simulink model "station"  (R2022a)
settings: Solver=VariableStepAuto  StartTime=0.0  StopTime=10.0  RelTol=1e-3
settings Model: Creator=kasturkoul  LastModifiedBy=kasturkoul

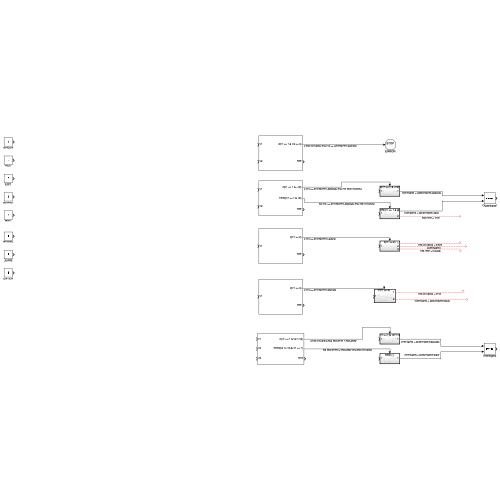
[thumbnail: Simulink's stored preview of the top-level diagram]
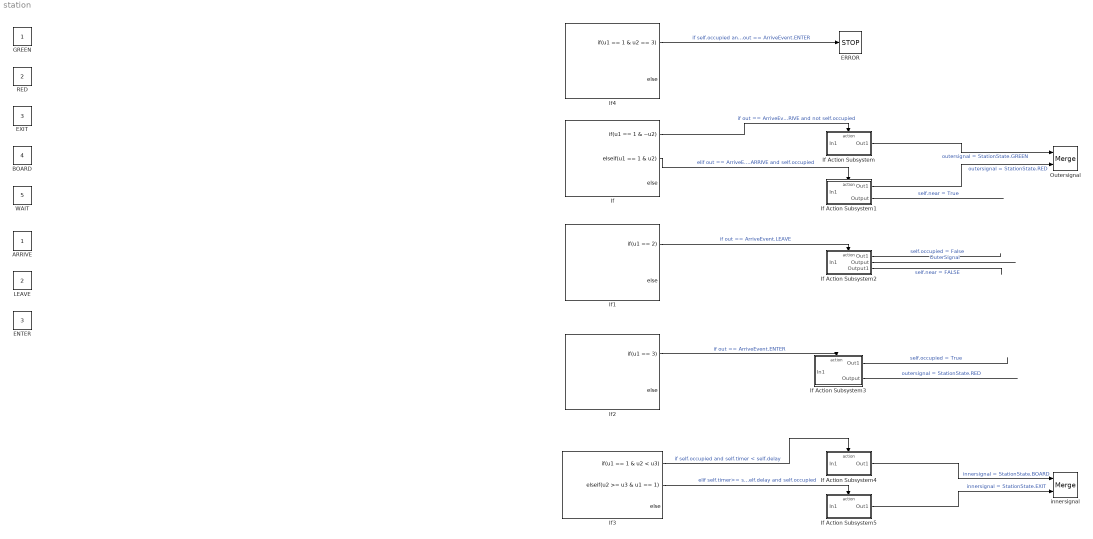
== system station ==
  ARRIVE : Constant
  BOARD : Constant  Value=4
  ENTER : Constant  Value=3
  ERROR : Stop
  EXIT : Constant  Value=3
  GREEN : Constant
  If : If  NumInputs=2  IfExpression=u1 == 1 & ~u2  ElseIfExpressions=u1 == 1 & u2
  If Action Subsystem : Subsystem  TreatAsAtomicUnit=on
  If Action Subsystem1 : Subsystem  TreatAsAtomicUnit=on
  If Action Subsystem2 : Subsystem  TreatAsAtomicUnit=on
  If Action Subsystem3 : Subsystem  TreatAsAtomicUnit=on
  If Action Subsystem4 : Subsystem  TreatAsAtomicUnit=on
  If Action Subsystem5 : Subsystem  TreatAsAtomicUnit=on
  If1 : If  IfExpression=u1 == 2
  If2 : If  IfExpression=u1 == 3
  If3 : If  NumInputs=3  IfExpression=u1 == 1 & u2 < u3  ElseIfExpressions=u2 >= u3 & u1 == 1
  If4 : If  NumInputs=2  IfExpression=u1 == 1 & u2 == 3
  LEAVE : Constant  Value=2
  Outersignal : Merge
  RED : Constant  Value=2
  WAIT : Constant  Value=5
  innersignal : Merge
  wires:
  If/1 -> If Action Subsystem/Action  "if out == ArriveEvent.ARRIVE and not self.occupied"
  If/2 -> If Action Subsystem1/Action  "elif out == ArriveEvent.ARRIVE and self.occupied"
  If1/1 -> If Action Subsystem2/Action  "if out == ArriveEvent.LEAVE"
  If2/1 -> If Action Subsystem3/Action  "if out == ArriveEvent.ENTER"
  If3/1 -> If Action Subsystem4/Action  "if self.occupied and self.timer < self.delay"
  If3/2 -> If Action Subsystem5/Action  "elif self.timer>= self.delay and self.occupied"
  If4/1 -> ERROR/1  "if self.occupied and out == ArriveEvent.ENTER"
  If Action Subsystem/1(Out1) -> Outersignal/1  "outersignal = StationState.GREEN"
  If Action Subsystem1/2(Output) -> ?  "self.near = True"
  If Action Subsystem1/1(Out1) -> Outersignal/2  "outersignal = StationState.RED"
  If Action Subsystem2/1(Out1) -> ?  "self.occupied = False"
  If Action Subsystem2/2(Output) -> ?  "OuterSignal"
  If Action Subsystem2/3(Output1) -> ?  "self.near = FALSE"
  If Action Subsystem3/2(Output) -> ?  "outersignal = StationState.RED"
  If Action Subsystem3/1(Out1) -> ?  "self.occupied = True"
  If Action Subsystem4/1(Out1) -> innersignal/1  "innersignal = StationState.BOARD"
  If Action Subsystem5/1(Out1) -> innersignal/2  "innersignal = StationState.EXIT"

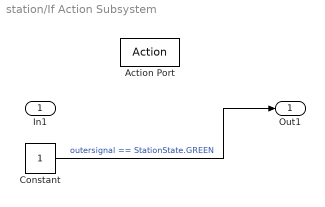
== system station/If Action Subsystem ==
  In1 : Inport
  Action Port : ActionPort  ActionPortLabel=if(u1 == 1 & ~u2)
  Constant : Constant
  Out1 : Outport
  wires:
  Constant/1 -> Out1/1  "outersignal == StationState.GREEN"

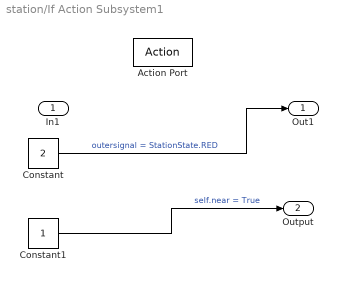
== system station/If Action Subsystem1 ==
  In1 : Inport
  Action Port : ActionPort  ActionPortLabel=elseif(u1 == 1 & u2)
  Constant : Constant  Value=2
  Constant1 : Constant
  Out1 : Outport
  Output : Outport  Port=2
  wires:
  Constant/1 -> Out1/1  "outersignal = StationState.RED"
  Constant1/1 -> Output/1  "self.near = True"

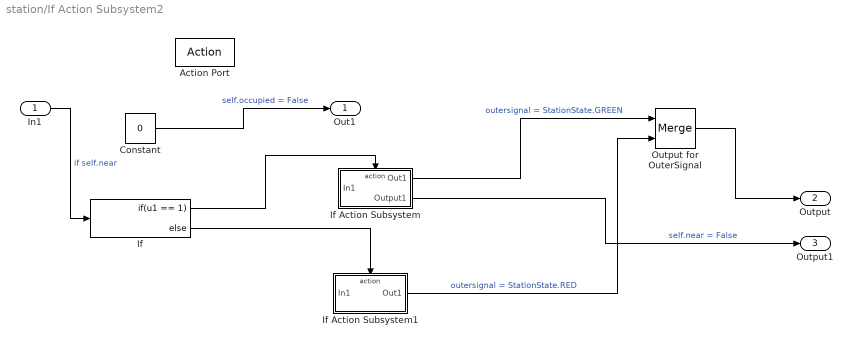
== system station/If Action Subsystem2 ==
  In1 : Inport
  Action Port : ActionPort  ActionPortLabel=if(u1 == 2)
  Constant : Constant  Value=0
  If : If  IfExpression=u1 == 1
  If Action Subsystem : Subsystem  TreatAsAtomicUnit=on
  If Action Subsystem1 : Subsystem  TreatAsAtomicUnit=on
  Output for OuterSignal : Merge
  Out1 : Outport
  Output : Outport  Port=2
  Output1 : Outport  Port=3
  wires:
  Constant/1 -> Out1/1  "self.occupied = False"
  In1/1 -> If/1  "if self.near"
  If/1 -> If Action Subsystem/Action
  If/2 -> If Action Subsystem1/Action
  If Action Subsystem/2(Output1) -> Output1/1  "self.near = False"
  If Action Subsystem/1(Out1) -> Output for OuterSignal/1  "outersignal = StationState.GREEN"
  If Action Subsystem1/1(Out1) -> Output for OuterSignal/2  "outersignal = StationState.RED"
  Output for OuterSignal/1 -> Output/1

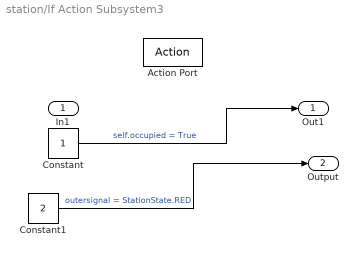
== system station/If Action Subsystem3 ==
  In1 : Inport
  Action Port : ActionPort  ActionPortLabel=if(u1 == 3)
  Constant : Constant
  Constant1 : Constant  Value=2
  Out1 : Outport
  Output : Outport  Port=2
  wires:
  Constant/1 -> Out1/1  "self.occupied = True"
  Constant1/1 -> Output/1  "outersignal = StationState.RED"

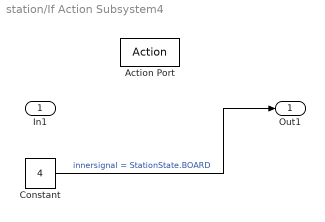
== system station/If Action Subsystem4 ==
  In1 : Inport
  Action Port : ActionPort  ActionPortLabel=if(u1 == 1 & u2 < u3)
  Constant : Constant  Value=4
  Out1 : Outport
  wires:
  Constant/1 -> Out1/1  "innersignal = StationState.BOARD"

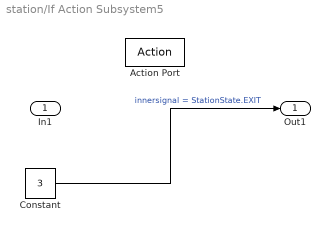
== system station/If Action Subsystem5 ==
  In1 : Inport
  Action Port : ActionPort  ActionPortLabel=elseif(u2 >= u3 & u1 == 1)
  Constant : Constant  Value=3
  Out1 : Outport
  wires:
  Constant/1 -> Out1/1  "innersignal = StationState.EXIT"

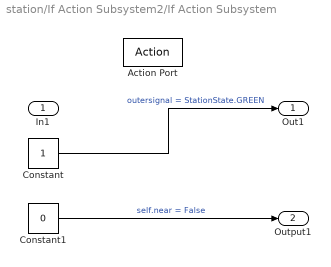
== system station/If Action Subsystem2/If Action Subsystem ==
  In1 : Inport
  Action Port : ActionPort  ActionPortLabel=if(u1 == 1)
  Constant : Constant
  Constant1 : Constant  Value=0
  Out1 : Outport
  Output1 : Outport  Port=2
  wires:
  Constant/1 -> Out1/1  "outersignal = StationState.GREEN"
  Constant1/1 -> Output1/1  "self.near = False"

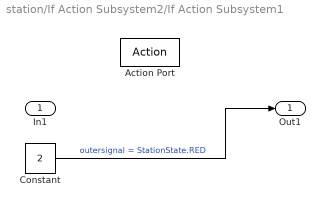
== system station/If Action Subsystem2/If Action Subsystem1 ==
  In1 : Inport
  Action Port : ActionPort  ActionPortLabel=else
  Constant : Constant  Value=2
  Out1 : Outport
  wires:
  Constant/1 -> Out1/1  "outersignal = StationState.RED"
